simulink model "ACC_Ver02_Operating_Modes"  (R2026a)
settings: Solver=FixedStepDiscrete  StopTime=inf  FixedStep=0.1
settings Model: Creator=Rakshith  LastModifiedBy=Rakshith

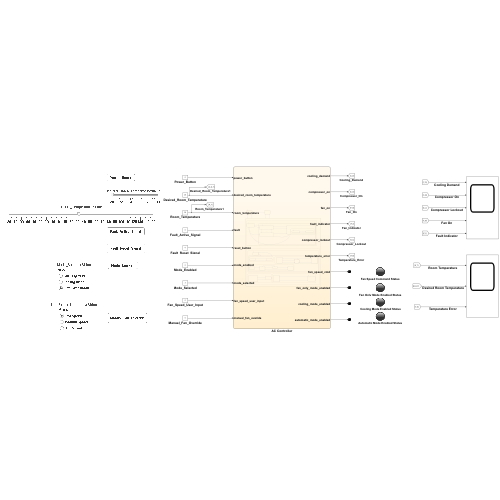
[thumbnail: Simulink's stored preview of the top-level diagram]
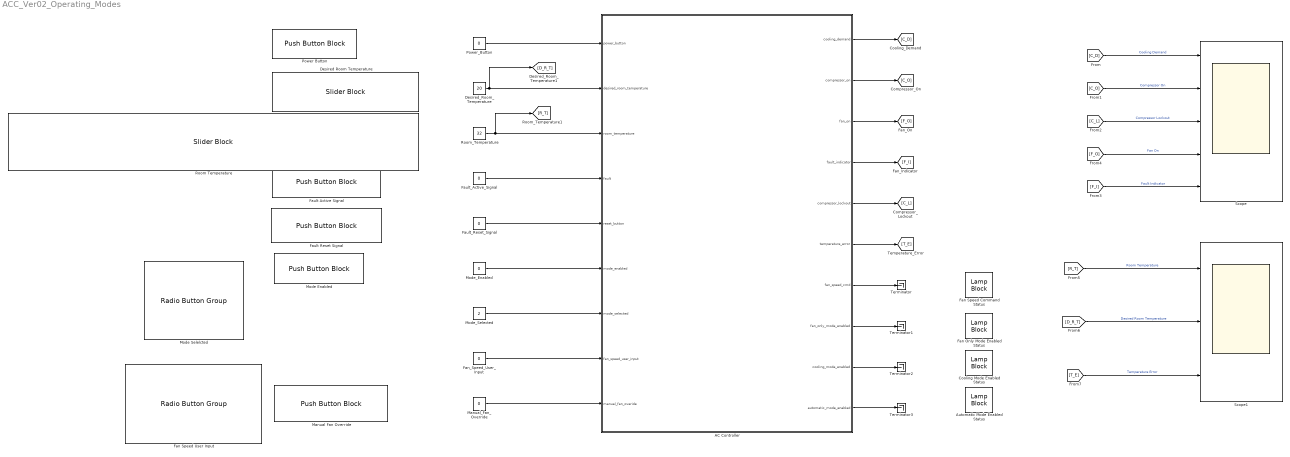
== system ACC_Ver02_Operating_Modes ==
  " Cooling Mode Enabled Status" : LampBlock  LabelPosition=Hide  DefaultColor=[0.0, 0.0, 0.0]
  AC Controller : Stateflow chart  TreatAsAtomicUnit=on
  Automatic Mode Enabled Status : LampBlock  LabelPosition=Hide  DefaultColor=[0.0, 0.0, 0.0]
  Desired Room Temperature : SliderBlock  ScaleMin=20  ScaleMax=30
  Desired_Room_Temperature : Constant  Value=20
  Fan Only Mode Enabled Status : LampBlock  LabelPosition=Hide  DefaultColor=[0.0, 0.0, 0.0]
  Fan Speed Command Status : LampBlock  LabelPosition=Hide  DefaultColor=[0.0, 0.0, 0.0]
  Fan Speed User Input : RadioButtonGroup  SelectedLabel=Low Speed  ButtonGroupName=Group
  Fan_Speed_User_Input : Constant  Value=0
  Fault Active Signal : PushButtonBlock  ButtonText=Fault_Active_Signal  ButtonType=Latch  IconOnColor=[0.0, 0.39215686274509803, 0.0]  IconOffColor=[0.0, 1.0, 0.0]  OffValue=0.000000
  Fault Reset Signal : PushButtonBlock  ButtonText=Fault_Reset_Signal  ButtonType=Latch  IconOnColor=[0.0, 0.39215686274509803, 0.0]  IconOffColor=[0.0, 1.0, 0.0]  OffValue=0.000000
  Fault_Active_Signal : Constant  Value=0
  Fault_Reset_Signal : Constant  Value=0
  Manual Fan Override : PushButtonBlock  ButtonText=Manual_Fan_Override  ButtonType=Latch  IconOnColor=[0.0, 0.39215686274509803, 0.0]  IconOffColor=[0.0, 1.0, 0.0]  OffValue=0.000000
  Manual_Fan_Override : Constant  Value=0
  Mode Enabled : PushButtonBlock  ButtonText=Mode_Enabled  ButtonType=Latch  IconOnColor=[0.0, 0.39215686274509803, 0.0]  IconOffColor=[0.0, 1.0, 0.0]  OffValue=0.000000
  Mode Selelcted : RadioButtonGroup  SelectedLabel=Automatic Mode  ButtonGroupName=Group
  Mode_Enabled : Constant  Value=0
  Mode_Selected : Constant  Value=2
  Power Button : PushButtonBlock  ButtonText=Power_Button  ButtonType=Latch  IconOnColor=[0.0, 0.39215686274509803, 0.0]  IconOffColor=[0.0, 1.0, 0.0]  OffValue=0.000000
  Power_Button : Constant  Value=0
  Room Temperature : SliderBlock  ScaleMin=-80  ScaleMax=150
  Room_Temperature : Constant  Value=32
  Scope : Scope  NumInputPorts=5
      settings: ActiveDisplayYMinimum=-0.12499999999999997  ActiveDisplayYMaximum=1.125
  Scope1 : Scope  NumInputPorts=3
      settings: ActiveDisplayYMinimum=22  ActiveDisplayYMaximum=42
  Terminator{,1..3} (4 alike) : Terminator
  wires:
  Fan_Speed_User_Input/1 -> AC Controller/8(fan_speed_user_input)
  [C_D] -> Scope/1  "Cooling Demand"
  Power_Button/1 -> AC Controller/1(power_button)
  AC Controller/4(fault_indicator) -> [F_I]
  AC Controller/2(compressor_on) -> [C_O]
  [C_O] -> Scope/2  "Compressor On"
  [C_L] -> Scope/3  "Compressor Lockout"
  [F_I] -> Scope/5  "Fault Indicator"
  Manual_Fan_Override/1 -> AC Controller/9(manual_fan_overide)
  AC Controller/1(cooling_demand) -> [C_D]
  [D_R_T] -> Scope1/2  "Desired Room Temperature"
  Fault_Active_Signal/1 -> AC Controller/4(fault)
  [T_E] -> Scope1/3  "Temperature Error"
  AC Controller/9(cooling_mode_enabled) -> Terminator2/1
  AC Controller/8(fan_only_mode_enabled) -> Terminator1/1
  AC Controller/7(fan_speed_cmd) -> Terminator/1
  Mode_Selected/1 -> AC Controller/7(mode_selected)
  [F_O] -> Scope/4  "Fan On"
  AC Controller/10(automatic_mode_enabled) -> Terminator3/1
  Mode_Enabled/1 -> AC Controller/6(mode_enabled)
  Fault_Reset_Signal/1 -> AC Controller/5(reset_button)
  Room_Temperature/1 -> AC Controller/3(room_temperature), [R_T]
  AC Controller/3(fan_on) -> [F_O]
  AC Controller/6(temperature_error) -> [T_E]
  AC Controller/5(compressor_lockout) -> [C_L]
  Desired_Room_Temperature/1 -> AC Controller/2(desired_room_temperature), [D_R_T]
  [R_T] -> Scope1/1  "Room Temperature"

== stateflow chart ACC_Ver02_Operating_Modes/AC Controller ==
  state Fault
    en: cooling_demand = 0;
    compressor_on = 0;
    compressor_lockout = 0;
    fan_on = 0;
    fan_speed_cmd = 0;
    fault_indicator = 1;
  state Power_Off
    en: cooling_demand = 0;
    compressor_on = 0;
    compressor_lockout = 0;
    fan_on = 0;
    fan_speed_cmd = 0;
    fault_indicator = 0;
  state Power_On
    en: fault_indicator = 0;
    du: set_temperature = desired_room_temperature; temperature_error = room_temperature-set_temperature;
    state Operating_Mode_Control [parallel]
      settings: executionOrder=2
      state Power_On_Standby
        en: cooling_control_enabled = 0;
        fan_only_mode_enabled = 0;
        cooling_mode_enabled = 0;
        automatic_mode_enabled = 0;
        automatic_fan_speed_enabled = 0;
        fan_speed_cmd = 1;
      state Power_On_Operating_Modes
        state Fan_Only_Mode
          en:cooling_control_enabled = 0;
          fan_only_mode_enabled = 1;
          cooling_mode_enabled = 0;
          automatic_mode_enabled = 0;
          automatic_fan_speed_enabled = 0;
          fan_speed_selected = fan_speed_user_input;
        state Automatic_Mode
          en: cooling_control_enabled = 1;
          fan_only_mode_enabled = 0;
          cooling_mode_enabled = 0;
          automatic_mode_enabled = 1;
          state Automatic_Mode_Fan_Speed_Source_Control [parallel]
            settings: executionOrder=1
            state Automatic_Fan_Speed_State
              en: automatic_fan_speed_enabled = 1;
            state Manual_Fan_Speed_Override_State
              en: automatic_fan_speed_enabled = 0;
            (default) -> Automatic_Fan_Speed_State
            Automatic_Fan_Speed_State -> Manual_Fan_Speed_Override_State : [ manual_fan_overide == 1 ]
            Manual_Fan_Speed_Override_State -> Automatic_Fan_Speed_State : [ manual_fan_overide == 0 ]
        state Cooling_Mode
          en:cooling_control_enabled = 1;
          fan_only_mode_enabled = 0;
          cooling_mode_enabled = 1;
          automatic_mode_enabled = 0;
          automatic_fan_speed_enabled = 0;
          fan_speed_selected = fan_speed_user_input;
        (default) -> Fan_Only_Mode
        Fan_Only_Mode -> Automatic_Mode [order 2] : [ mode_enabled == 1 && mode_selected == 2 ]
        Automatic_Mode -> Fan_Only_Mode [order 1] : [ mode_enabled == 1 && mode_selected == 0 ]
        Fan_Only_Mode -> Cooling_Mode [order 1] : [ mode_enabled == 1 && mode_selected == 1 ]
        Cooling_Mode -> Fan_Only_Mode [order 1] : [ mode_enabled == 1 && mode_selected == 0 ]
        Cooling_Mode -> Automatic_Mode [order 2] : [ mode_enabled == 1 && mode_selected == 2 ]
        Automatic_Mode -> Cooling_Mode [order 2] : [ mode_enabled == 1 && mode_selected == 1 ]
      (default) -> Power_On_Standby
      Power_On_Operating_Modes -> Power_On_Standby : [ mode_enabled == 0 ]
      Power_On_Standby -> Fan_Only_Mode [order 1] : [ mode_enabled == 1 && mode_selected == 0 ]
      Power_On_Standby -> Automatic_Mode [order 3] : [ mode_enabled == 1 && mode_selected == 2 ]
      Power_On_Standby -> Cooling_Mode [order 2] : [ mode_enabled == 1 && mode_selected == 1 ]
    state Cooling_Control_and_Fan_Speed_Control_Mechanism [parallel]
      settings: executionOrder=1
      state Cooling_Control_Mechanism [parallel]
        settings: executionOrder=1
        state Cooling_Control_Standby
          en: cooling_demand = 0;
          compressor_on = 0;
          compressor_lockout = 0;
          fan_on = 1;
        state Cooling_Control
          state Compressor_Mechanism [parallel]
            settings: executionOrder=1
            state Compressor_Activation
              en: compressor_on = 1;
              compressor_lockout = 0;
            state Compressor_Deactivation
              en: compressor_on = 0;
              compressor_lockout = 0;
            state Compressor_Lockout
              en: compressor_on = 0;
              compressor_lockout = 1;
            Compressor_Deactivation -> Compressor_Activation : [ cooling_demand ==1 ]
            (default) -> Compressor_Lockout
            Compressor_Lockout -> Compressor_Activation [order 1] : [ after(compressor_min_off_time, sec) && cooling_demand ==1 ]
            Compressor_Activation -> Compressor_Lockout : [ cooling_demand == 0 ]
            Compressor_Lockout -> Compressor_Deactivation [order 2] : [ after(compressor_min_off_time, sec) && cooling_demand == 0 ]
          state Cooling_Demand [parallel]
            settings: executionOrder=3
            state Cooling_Demand_Activation
              en: cooling_demand = 1;
            state Cooling_Demand_Deactivation
              en: cooling_demand = 0;
            (default) -> Cooling_Demand_Deactivation
            Cooling_Demand_Deactivation -> Cooling_Demand_Activation : [ temperature_error >= temperature_hysteresis_band ]
            Cooling_Demand_Activation -> Cooling_Demand_Deactivation : [ temperature_error <= -temperature_hysteresis_band ]
          state Fan_Mechanism [parallel]
            settings: executionOrder=2
            state Fan_Activation
              en: fan_on = 1;
            state Compressor_Off_Check
              en: fan_on = 1;
            state Fan_Deactivation
              en: fan_on = 0;
            state Fan_On_Standby
              en: fan_on = 1;
            Compressor_Off_Check -> Fan_Activation [order 1] : [ compressor_on == 1 ]
            (default) -> Fan_On_Standby
            Fan_Activation -> Compressor_Off_Check : [ compressor_on == 0 ]
            Compressor_Off_Check -> Fan_Deactivation [order 2] : [ after(fan_run_on_time, sec) && compressor_on == 0 ]
            Fan_On_Standby -> Fan_Activation : [ compressor_on == 1 ]
            Fan_Deactivation -> Fan_Activation : [ compressor_on == 1 ]
        (default) -> Cooling_Control_Standby
        Cooling_Control -> Cooling_Control_Standby : [ cooling_control_enabled == 0 ]
        Cooling_Control_Standby -> Cooling_Control : [ cooling_control_enabled == 1 ]
      state Manual_Fan_Speed_Selection [parallel]
        settings: executionOrder=3
        state Manual_Fan_Speed_Logic
          du:
          if fan_on == 0
          fan_speed_cmd = 0;
          elseif fan_speed_user_input == 0
          fan_speed_cmd = 1;
          elseif fan_speed_user_input == 1
          fan_speed_cmd = 2;
          elseif fan_speed_user_input == 2
          fan_speed_cmd = 3
          else
          fan_speed_cmd = 1;
          end
        state Manual_Fan_Speed_Standby
        (default) -> Manual_Fan_Speed_Standby
        Manual_Fan_Speed_Standby -> Manual_Fan_Speed_Logic : [ (fan_only_mode_enabled == 1 || cooling_mode_enabled == 1 || automatic_mode_enabled == 1) && automatic_fan_speed_enabled == 0 ]
        Manual_Fan_Speed_Logic -> Manual_Fan_Speed_Standby : [ (fan_only_mode_enabled == 0 && cooling_mode_enabled == 0 && automatic_mode_enabled == 0) ||  automatic_fan_speed_enabled == 1 ]
      state Automatic_Fan_Speed_Selection [parallel]
        settings: executionOrder=2
        state Automatic_Fan_Speed_Logic
          du:
          if fan_on == 0
          fan_speed_cmd = 0;
          elseif compressor_on == 0
          fan_speed_cmd = 1;
          elseif temperature_error < medium_speed_threshold
          fan_speed_cmd = 1;
          elseif temperature_error < high_speed_threshold
          fan_speed_cmd = 2;
          else
          fan_speed_cmd = 3;
          end
        state Automatic_Fan_Speed_Standby
        (default) -> Automatic_Fan_Speed_Standby
        Automatic_Fan_Speed_Standby -> Automatic_Fan_Speed_Logic : [ automatic_fan_speed_enabled == 1 ]
        Automatic_Fan_Speed_Logic -> Automatic_Fan_Speed_Standby : [ automatic_fan_speed_enabled == 0 ]
  (default) -> Power_Off
  Fault -> Power_Off [order 2] : [ ( reset_button == 1 && fault == 0 ) && power_button == 0 ]
  Fault -> Power_On [order 1] : [ ( reset_button == 1 && fault == 0 ) && power_button == 1 ]
  Power_On -> Fault [order 1] : [ fault == 1 ]
  Power_Off -> Power_On : [ power_button == 1 ]
  Power_On -> Power_Off [order 2] : [ power_button == 0 ]
  data: cooling_demand output; compressor_on output; fan_on output; fault_indicator output; compressor_lockout output; temperature_error output; power_button input; compressor_min_off_time local =15; desired_room_temperature input; room_temperature input; fault input; reset_button input; mode_enabled input; mode_selected input; fan_run_on_time local =120; fan_speed_user_input input; high_speed_threshold local =15; manual_fan_overide input; medium_speed_threshold local =10; temperature_hysteresis_band local =7.5; fan_speed_cmd output; automatic_fan_speed_enabled local =0; cooling_control_enabled local =0; set_temperature local =0; fan_speed_selected local =0; fan_only_mode_enabled output; cooling_mode_enabled output; automatic_mode_enabled output
